simulink model "DCmodel_controlled_AWU_FFC_OLD"  (R2020b)
settings: Solver=VariableStepAuto  StartTime=0.0  StopTime=3  FixedStep=0.001  RelTol=1e-3
values from neighbouring files (symbols this model uses):
  B_eq = 1.08274338039e-06    [DIGIT1-BE20.mat]    (also in DIGIT1-BE4.mat; DIGIT1-TR4.mat; P2FFUOFF.mat; load_params_inertial_case.m = LSopt(1))
  degs2rpm = 0.166666666667    [DIGIT1-BE20.mat]    (also in DIGIT1-BE4.mat; DIGIT1-TR4.mat; P2FFUOFF.mat; load_params_inertial_case.m)
  drv =     [DIGIT1-BE20.mat]    (also in DIGIT1-BE4.mat; DIGIT1-TR4.mat; P2FFUOFF.mat)
  filt =     [DIGIT1-BE20.mat]    (also in DIGIT1-BE4.mat; DIGIT1-TR4.mat; P2FFUOFF.mat)
  gbox =     [DIGIT1-BE20.mat]    (also in DIGIT1-BE4.mat; DIGIT1-TR4.mat; P2FFUOFF.mat)
  J_eq = 7.3238e-07    [DIGIT1-BE20.mat]    (also in DIGIT1-BE4.mat; DIGIT1-TR4.mat; P2FFUOFF.mat; load_params_inertial_case.m = LSopt(3))
  mld =     [DIGIT1-BE20.mat]    (also in DIGIT1-BE4.mat; DIGIT1-TR4.mat; P2FFUOFF.mat)
  mot =     [DIGIT1-BE20.mat]    (also in DIGIT1-BE4.mat; DIGIT1-TR4.mat; P2FFUOFF.mat)
  rads2rpm = 9.54929658551    [DIGIT1-BE20.mat]    (also in DIGIT1-BE4.mat; DIGIT1-TR4.mat; P2FFUOFF.mat; load_params_inertial_case.m)
  rpm2rads = 0.10471975512    [DIGIT1-BE20.mat]    (also in DIGIT1-BE4.mat; DIGIT1-TR4.mat; P2FFUOFF.mat; load_params_inertial_case.m)
  sens =     [DIGIT1-BE20.mat]    (also in DIGIT1-BE4.mat; DIGIT1-TR4.mat; P2FFUOFF.mat)
  tausf = 0.0098    [DIGIT1-BE20.mat]    (also in DIGIT1-BE4.mat; DIGIT1-TR4.mat; P2FFUOFF.mat; load_params_inertial_case.m = LSopt(2))
libraries: simulink x1
settings Model: Creator=emanuelevitetta  LastModifiedBy=verrimarco
settings SolverCC: ZeroCrossAlgorithm=Adaptive
settings DebuggingCC: IgnoredZcDiagnostic=none  SFMachineParentedDataDiag=error

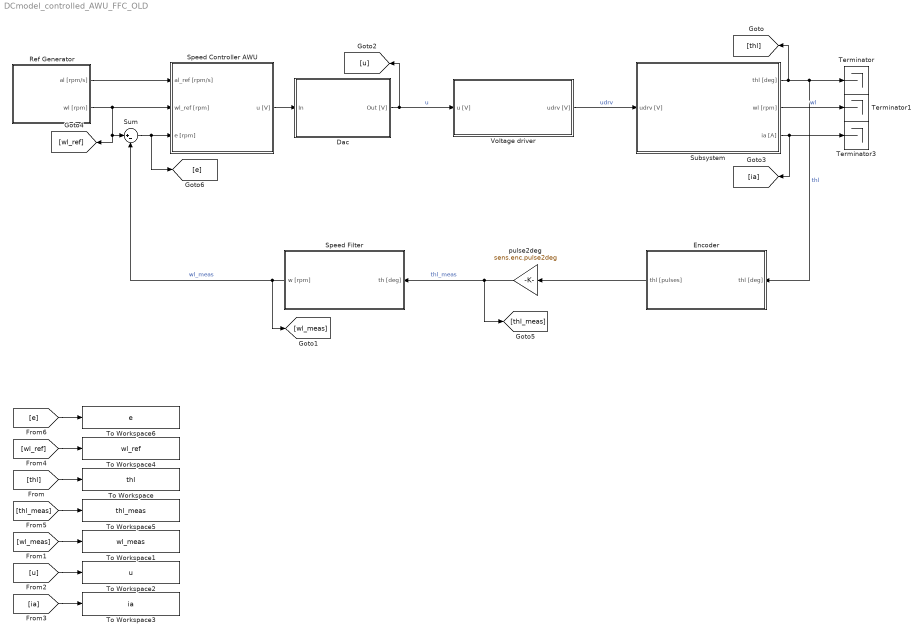
== system DCmodel_controlled_AWU_FFC_OLD ==
  Dac : Subsystem
  Encoder : Subsystem
  Ref Generator : Subsystem
  Speed Controller AWU : Subsystem
  Speed Filter : Subsystem
  Subsystem : Subsystem
  Sum : Sum  Inputs=|+-
  Terminator : Terminator
  Terminator1 : Terminator
  Terminator3 : Terminator
  To Workspace : ToWorkspace  VariableName=thl  SaveFormat=Timeseries  SampleTime=-1
      settings: Save2DSignal=2-D array (concatenate along first dimension)
  To Workspace1 : ToWorkspace  VariableName=wl_meas  SaveFormat=Timeseries  SampleTime=-1
      settings: Save2DSignal=2-D array (concatenate along first dimension)
  To Workspace2 : ToWorkspace  VariableName=u  SaveFormat=Timeseries  SampleTime=-1
      settings: Save2DSignal=2-D array (concatenate along first dimension)
  To Workspace3 : ToWorkspace  VariableName=ia  SaveFormat=Timeseries  SampleTime=-1
      settings: Save2DSignal=2-D array (concatenate along first dimension)
  To Workspace4 : ToWorkspace  VariableName=wl_ref  SaveFormat=Timeseries  SampleTime=-1
      settings: Save2DSignal=2-D array (concatenate along first dimension)
  To Workspace5 : ToWorkspace  VariableName=thl_meas  SaveFormat=Timeseries  SampleTime=-1
      settings: Save2DSignal=2-D array (concatenate along first dimension)
  To Workspace6 : ToWorkspace  VariableName=e  SaveFormat=Timeseries  SampleTime=-1
      settings: Save2DSignal=2-D array (concatenate along first dimension)
  Voltage driver : Subsystem
  pulse2deg : Gain  Gain=sens.enc.pulse2deg
  wires:
  Dac/1(Out [V]) -> [u], Voltage driver/1(u [V])  "u"
  Encoder/1(thl [pulses]) -> pulse2deg/1
  Voltage driver/1(udrv [V]) -> Subsystem/1(udrv [V])  "udrv"
  Subsystem/2(wl [rpm]) -> Terminator1/1  "wl"
  Subsystem/1(thl [deg]) -> Terminator/1, Encoder/1(thl [deg]), [thl]  "thl"
  pulse2deg/1 -> [thl_meas], Speed Filter/1(th [deg])  "thl_meas"
  Speed Filter/1(w [rpm]) -> Sum/2, [wl_meas]  "wl_meas"
  Subsystem/3(ia [A]) -> Terminator3/1, [ia]
  [thl] -> To Workspace/1
  [wl_meas] -> To Workspace1/1
  [ia] -> To Workspace3/1
  [u] -> To Workspace2/1
  [wl_ref] -> To Workspace4/1
  [thl_meas] -> To Workspace5/1
  Sum/1 -> [e], Speed Controller AWU/3(e [rpm])
  Speed Controller AWU/1(u [V]) -> Dac/1(In)
  [e] -> To Workspace6/1
  Ref Generator/1(al [rpm/s]) -> Speed Controller AWU/1(al_ref [rpm/s])
  Ref Generator/2(wl [rpm]) -> [wl_ref], Sum/1, Speed Controller AWU/2(wl_ref [rpm])

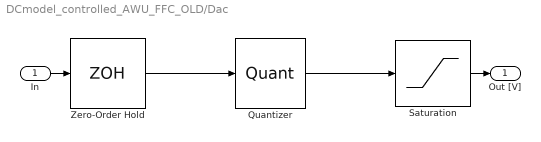
== system DCmodel_controlled_AWU_FFC_OLD/Dac ==
  In : Inport
  Quantizer : Quantizer  QuantizationInterval=daq.dac.q
  Saturation : Saturate  UpperLimit=10  LowerLimit=-10
  Zero-Order Hold : ZeroOrderHold  SampleTime=0.001
  Out [V] : Outport
  wires:
  In/1 -> Zero-Order Hold/1
  Zero-Order Hold/1 -> Quantizer/1
  Saturation/1 -> Out [V]/1
  Quantizer/1 -> Saturation/1

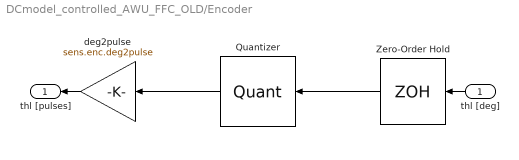
== system DCmodel_controlled_AWU_FFC_OLD/Encoder ==
  thl [deg] : Inport
  Quantizer : Quantizer  QuantizationInterval=sens.enc.pulse2deg
  Zero-Order Hold : ZeroOrderHold  SampleTime=0.001
  deg2pulse : Gain  Gain=sens.enc.deg2pulse
  thl [pulses] : Outport
  wires:
  deg2pulse/1 -> thl [pulses]/1
  Quantizer/1 -> deg2pulse/1
  thl [deg]/1 -> Zero-Order Hold/1
  Zero-Order Hold/1 -> Quantizer/1

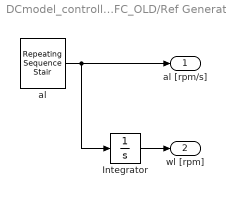
== system DCmodel_controlled_AWU_FFC_OLD/Ref Generator ==
  Integrator : Integrator
  al : simulink/Sources/Repeating Sequence Stair  OutValues=[900 0 -900 -900 0 900].'  tsamp=0.5  OutMin=[]  OutMax=[]  OutDataTypeStr=double  OutputDataTypeScalingMode=double  OutDataType=fixdt(0,8)  ConRadixGroup=Best Precision: Vector-wise  OutScaling=2^-12
  al [rpm/s] : Outport
  wl [rpm] : Outport  Port=2
  wires:
  al/1 -> Integrator/1, al [rpm/s]/1
  Integrator/1 -> wl [rpm]/1

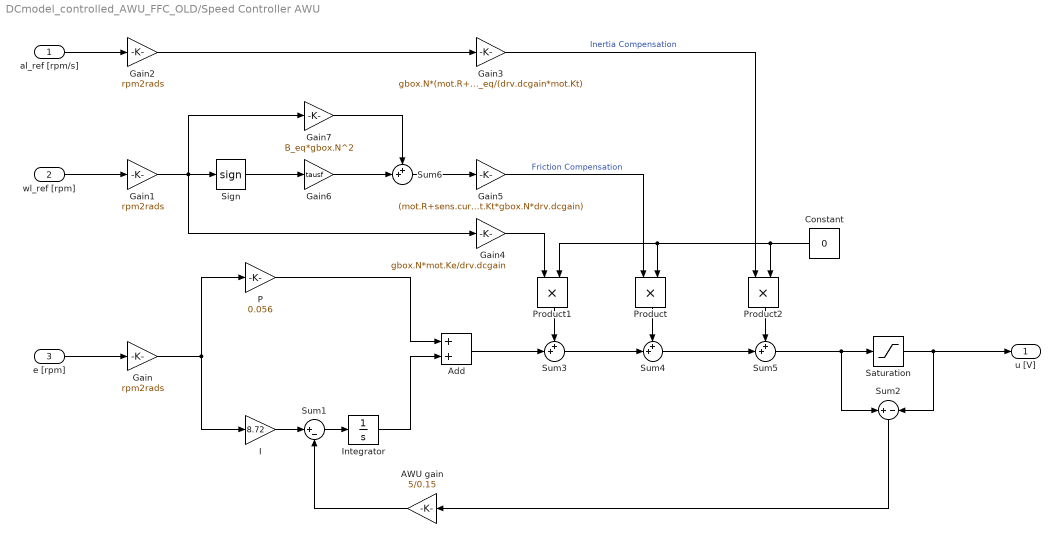
== system DCmodel_controlled_AWU_FFC_OLD/Speed Controller AWU ==
  al_ref [rpm/s] : Inport
  wl_ref [rpm] : Inport  Port=2
  e [rpm] : Inport  Port=3
  AWU gain : Gain  Gain=5/0.15
  Add : Sum
  Constant : Constant  Value=0
  Gain : Gain  Gain=rpm2rads
  Gain1 : Gain  Gain=rpm2rads
  Gain2 : Gain  Gain=rpm2rads
  Gain3 : Gain  Gain=gbox.N*(mot.R+sens.curr.Rs)*J_eq/(drv.dcgain*mot.Kt)
  Gain4 : Gain  Gain=gbox.N*mot.Ke/drv.dcgain
  Gain5 : Gain  Gain=(mot.R+sens.curr.Rs)/(mot.Kt*gbox.N*drv.dcgain)
  Gain6 : Gain  Gain=tausf
  Gain7 : Gain  Gain=B_eq*gbox.N^2
  I : Gain  Gain=8.72
  Integrator : Integrator
  P : Gain  Gain=0.056
  Product : Product
  Product1 : Product
  Product2 : Product
  Saturation : Saturate  UpperLimit=10  LowerLimit=-10
  Sign : Signum
  Sum1 : Sum  Inputs=|+-
  Sum2 : Sum  Inputs=+-
  Sum{3..6} (4 alike) : Sum  Inputs=++|
  u [V] : Outport
  wires:
  e [rpm]/1 -> Gain/1
  P/1 -> Add/1
  Integrator/1 -> Add/2
  Saturation/1 -> Sum2/2, u [V]/1
  Gain/1 -> I/1, P/1
  Sum1/1 -> Integrator/1
  I/1 -> Sum1/1
  Sum2/1 -> AWU gain/1
  AWU gain/1 -> Sum1/2
  wl_ref [rpm]/1 -> Gain1/1
  al_ref [rpm/s]/1 -> Gain2/1
  Gain2/1 -> Gain3/1
  Sum6/1 -> Gain5/1
  Gain6/1 -> Sum6/2
  Gain5/1 -> Product/1  "Friction Compensation"
  Gain3/1 -> Product2/1  "Inertia Compensation"
  Gain4/1 -> Product1/1
  Sign/1 -> Gain6/1
  Gain1/1 -> Gain4/1, Gain7/1, Sign/1
  Gain7/1 -> Sum6/1
  Add/1 -> Sum3/2
  Sum3/1 -> Sum4/2
  Sum4/1 -> Sum5/2
  Sum5/1 -> Sum2/1, Saturation/1
  Product1/1 -> Sum3/1
  Product/1 -> Sum4/1
  Product2/1 -> Sum5/1
  Constant/1 -> Product2/2, Product/2, Product1/2

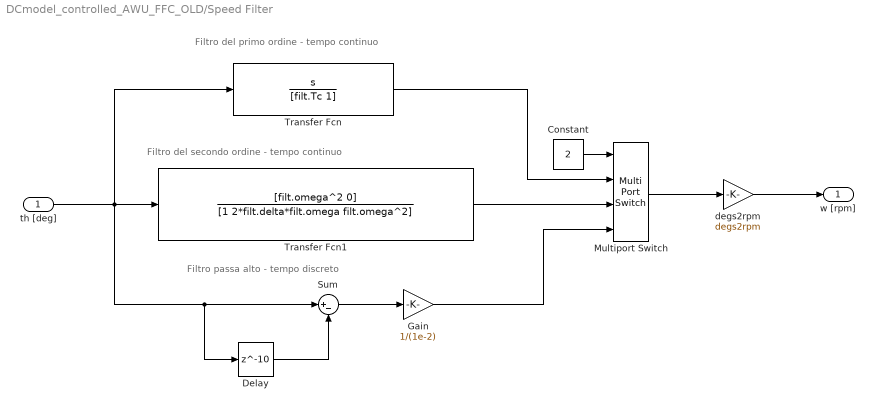
== system DCmodel_controlled_AWU_FFC_OLD/Speed Filter ==
  note: Filtro passa alto - tempo discreto
  note: Filtro del secondo ordine - tempo continuo
  note: Filtro del primo ordine - tempo continuo
  th [deg] : Inport
  Constant : Constant  Value=2
  Delay : Delay  DelayLength=10  InitialCondition=0
  Gain : Gain  Gain=1/(1e-2)
  Multiport Switch : MultiPortSwitch
  Sum : Sum  Inputs=|+-
  Transfer Fcn : TransferFcn  Numerator=[1 0]  Denominator=[filt.Tc 1]
  Transfer Fcn1 : TransferFcn  Numerator=[filt.omega^2 0]  Denominator=[1 2*filt.delta*filt.omega filt.omega^2]
  degs2rpm : Gain  Gain=degs2rpm
  w [rpm] : Outport
  wires:
  degs2rpm/1 -> w [rpm]/1
  Transfer Fcn1/1 -> Multiport Switch/3
  Multiport Switch/1 -> degs2rpm/1
  Gain/1 -> Multiport Switch/4
  Delay/1 -> Sum/2
  Sum/1 -> Gain/1
  Constant/1 -> Multiport Switch/1
  Transfer Fcn/1 -> Multiport Switch/2
  th [deg]/1 -> Delay/1, Sum/1, Transfer Fcn/1, Transfer Fcn1/1

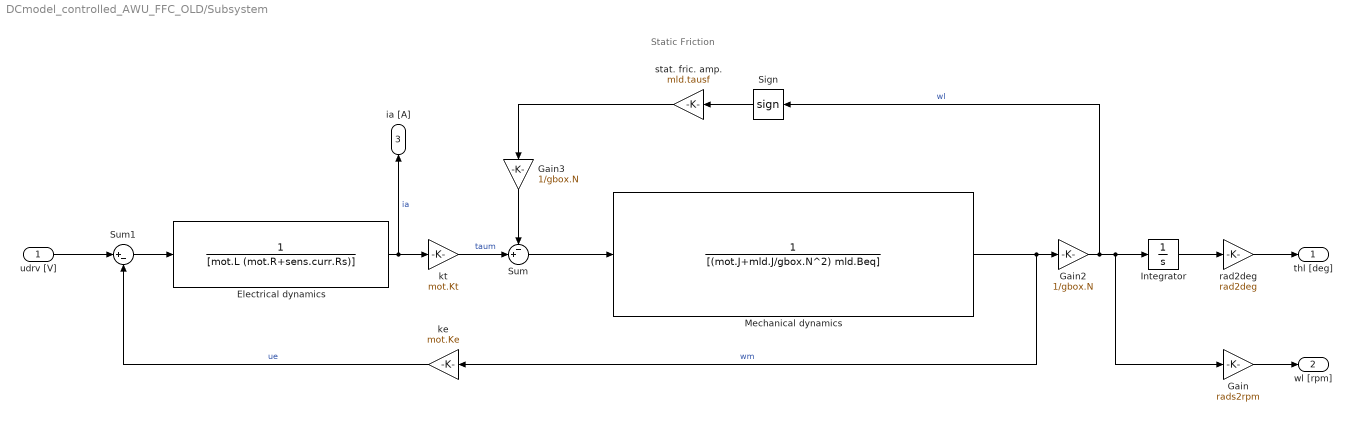
== system DCmodel_controlled_AWU_FFC_OLD/Subsystem ==
  note: Static Friction
  udrv [V] : Inport
  Electrical dynamics : TransferFcn  Denominator=[mot.L (mot.R+sens.curr.Rs)]
  Gain : Gain  Gain=rads2rpm
  Gain2 : Gain  Gain=1/gbox.N
  Gain3 : Gain  Gain=1/gbox.N
  Integrator : Integrator
  Mechanical dynamics : TransferFcn  Denominator=[(mot.J+mld.J/gbox.N^2) mld.Beq]
  Sign : Signum
  Sum : Sum  Inputs=-+|
  Sum1 : Sum  Inputs=|+-
  ke : Gain  Gain=mot.Ke
  kt : Gain  Gain=mot.Kt
  rad2deg : Gain  Gain=rad2deg
  stat. fric. amp. : Gain  Gain=mld.tausf
  thl [deg] : Outport
  wl [rpm] : Outport  Port=2
  ia [A] : Outport  Port=3
  wires:
  rad2deg/1 -> thl [deg]/1
  Integrator/1 -> rad2deg/1
  Gain/1 -> wl [rpm]/1
  kt/1 -> Sum/2  "taum"
  Sum/1 -> Mechanical dynamics/1
  Electrical dynamics/1 -> kt/1, ia [A]/1  "ia"
  Mechanical dynamics/1 -> ke/1, Gain2/1  "wm"
  Gain2/1 -> Sign/1, Gain/1, Integrator/1  "wl"
  Sign/1 -> stat. fric. amp./1
  stat. fric. amp./1 -> Gain3/1
  Sum1/1 -> Electrical dynamics/1
  ke/1 -> Sum1/2  "ue"
  udrv [V]/1 -> Sum1/1
  Gain3/1 -> Sum/1

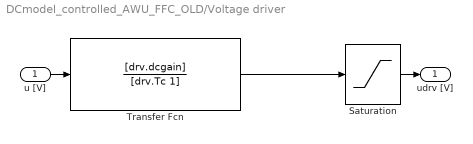
== system DCmodel_controlled_AWU_FFC_OLD/Voltage driver ==
  u [V] : Inport
  Saturation : Saturate  UpperLimit=12  LowerLimit=-12
  Transfer Fcn : TransferFcn  Numerator=[drv.dcgain]  Denominator=[drv.Tc 1]
  udrv [V] : Outport
  wires:
  u [V]/1 -> Transfer Fcn/1
  Saturation/1 -> udrv [V]/1
  Transfer Fcn/1 -> Saturation/1
